simulink model "2_5285361396970701638"  (R2023b)
settings: Solver=VariableStepAuto  StartTime=0.0  StopTime=30  RelTol=1e-3
libraries: simulink x2
settings Model: SimulationMode=accelerator  Creator=ermol  LastModifiedBy=ermol

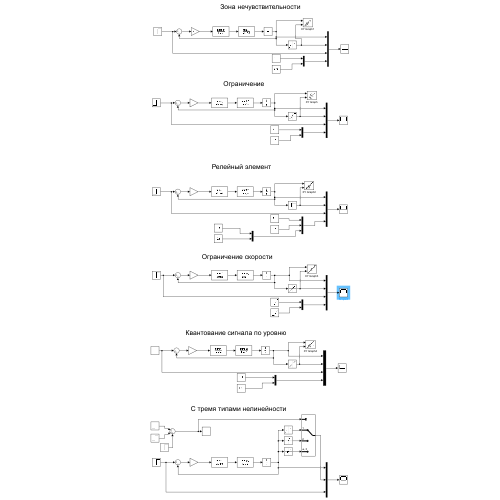
[thumbnail: Simulink's stored preview of the top-level diagram]
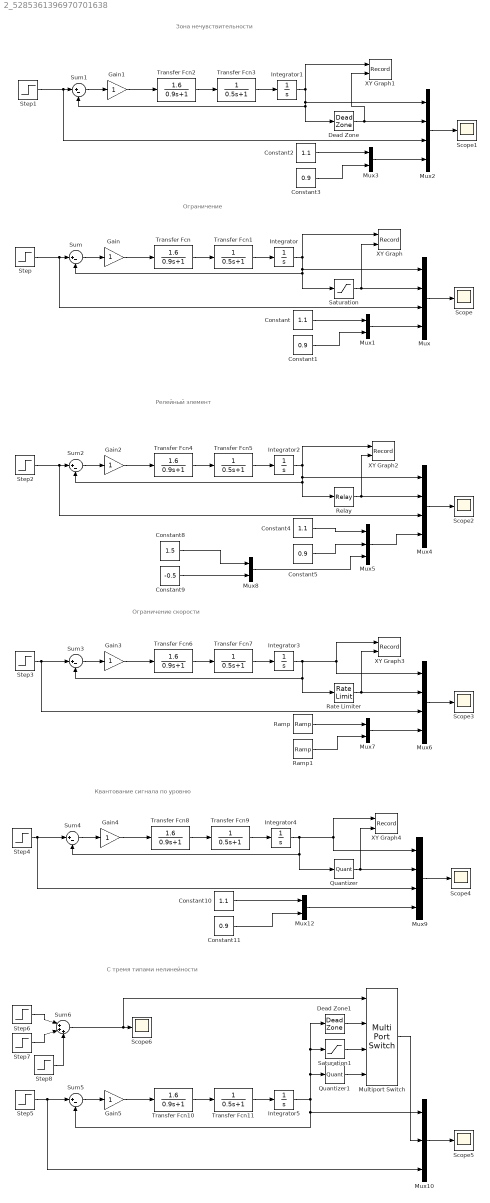
== system 2_5285361396970701638 ==
  note: Ограничение
  note: Зона нечувствительности
  note: Релейный элемент
  note: Ограничение скорости
  note: Квантование сигнала по уровню
  note: С тремя типами нелинейности
  Constant{,2,4,10} (4 alike) : Constant  Value=1.1
  Constant{1,3,5,11} (4 alike) : Constant  Value=0.9
  Constant8 : Constant  Value=1.5
  Constant9 : Constant  Value=-0.5
  Dead Zone : DeadZone  LowerValue=0.9  UpperValue=1.1
  Dead Zone1 : DeadZone  LowerValue=0.9  UpperValue=1.1
  Gain{,1..5} (6 alike) : Gain
  Integrator{,1..5} (6 alike) : Integrator
  Multiport Switch : MultiPortSwitch  SaturateOnIntegerOverflow=off  InputSameDT=off
  Mux{,2,4,6,9} (5 alike) : Mux
  Mux{1,3,7..8,12} (5 alike) : Mux  Inputs=2
  Mux10 : Mux  Inputs=3
  Mux5 : Mux  Inputs=3
  Quantizer : Quantizer  QuantizationInterval=0.2
  Quantizer1 : Quantizer  QuantizationInterval=0.2
  Ramp : simulink/Sources/Ramp  slope=0.3  start=0  InitialOutput=0
  Ramp1 : simulink/Sources/Ramp  slope=-0.15  start=0  InitialOutput=0
  Rate Limiter : RateLimiter  RisingSlewLimit=0.3  FallingSlewLimit=-0.15  SampleTimeMode=inherited
  Relay : Relay  OnSwitchValue=1.1  OffSwitchValue=0.9  OnOutputValue=1.5  OffOutputValue=-0.5
  Saturation : Saturate  UpperLimit=1.1  LowerLimit=0.9
  Saturation1 : Saturate  UpperLimit=1.1  LowerLimit=0.9
  Scope{,1..6} (7 alike) : Scope
  Step{,1..6} (7 alike) : Step  Time=0  SampleTime=0
  Step7 : Step  Time=10  SampleTime=0
  Step8 : Step  Time=20  SampleTime=0
  Sum{,1..5} (6 alike) : Sum  Inputs=|+-
  Sum6 : Sum  Inputs=|+++
  Transfer Fcn{,2,4,6,8,10} (6 alike) : TransferFcn  Numerator=[1.6]  Denominator=[0.9 1]
  Transfer Fcn{1,3,5,7,9,11} (6 alike) : TransferFcn  Denominator=[0.5 1]
  XY Graph : Record  FileSettingsInternal="{\"entries\":[{\"content\":{\"excelSettings\":{\"content\":{},\"type\":\"Streamout.ExcelSettings\"}},\"type\":\"Streamout.FileSettingStorage\",\"uuid\":\"\"}],\"packageUris\":[\"http:\\/\\/schema.mathworks.com\\/mf0\\/streamout_blocks\\/R2020a\"],\"version\":\"1.0\"}"  Layout=[1 1]  SignalsInternal="{\"entries\":[{\"content\":{\"signals\":[{\"content\":{\"blockPath\":[],\"dimensions\":[1],\"domain\":\"\",\"lineColor\":\"#a2142f\",\"plots\":[1],\"port\":1,\"sid\":[\"\"],\"signalID\":2000,\"signalName\":\"Integrator\"},\"type\":\"RecordBlkView.Signal\",\"uuid\":\"\"},{\"content\":{\"blockPath\":[],\"dimensions\":[1],\"domain\":\"\",\"lineColor\":\"#139fff\",\"plots\":[1],\"port\":2,\"sid\":[\"\"],\"signalID\":2004,\"signalName\":\"Saturation\"},\"type\":\"RecordBlkView.Signal\",\"uuid\":\"\"}]},\"type\":\"RecordBlkView.InputSignals\",\"uuid\":\"\"}],\"packageUris\":[\"http:\\/\\/schema.mathworks.com\\/mf0\\/streamout_blocks\\/R2020a\"],\"version\":\"1.0\"}"  VisualizationBindings="{\"xyplotplugin\":{\"info\":[{\"series\":[{\"bindingParametersList\":[{\"parameter\":\"X-Axis\",\"signalID\":2000,\"signalName\":\"Integrator\"},{\"parameter\":\"Y-Axis\",\"signalID\":2004,\"signalName\":\"Saturation\"}],\"seriesID\":16176}],\"subplotID\":1}]}}"  CompatibilityTag=XY
  XY Graph1 : Record  FileSettingsInternal="{\"entries\":[{\"content\":{\"excelSettings\":{\"content\":{},\"type\":\"Streamout.ExcelSettings\"}},\"type\":\"Streamout.FileSettingStorage\",\"uuid\":\"\"}],\"packageUris\":[\"http:\\/\\/schema.mathworks.com\\/mf0\\/streamout_blocks\\/R2020a\"],\"version\":\"1.0\"}"  Layout=[1 1]  SignalsInternal="{\"entries\":[{\"content\":{\"signals\":[{\"content\":{\"blockPath\":[],\"dimensions\":[1],\"domain\":\"\",\"lineColor\":\"#a2142f\",\"plots\":[1],\"port\":1,\"sid\":[\"\"],\"signalID\":2016,\"signalName\":\"Integrator1\"},\"type\":\"RecordBlkView.Signal\",\"uuid\":\"\"},{\"content\":{\"blockPath\":[],\"dimensions\":[1],\"domain\":\"\",\"lineColor\":\"#139fff\",\"plots\":[1],\"port\":2,\"sid\":[\"\"],\"signalID\":2020,\"signalName\":\"Dead Zone\"},\"type\":\"RecordBlkView.Signal\",\"uuid\":\"\"}]},\"type\":\"RecordBlkView.InputSignals\",\"uuid\":\"\"}],\"packageUris\":[\"http:\\/\\/schema.mathworks.com\\/mf0\\/streamout_blocks\\/R2020a\"],\"version\":\"1.0\"}"  VisualizationBindings="{\"xyplotplugin\":{\"info\":[{\"series\":[{\"bindingParametersList\":[{\"parameter\":\"X-Axis\",\"signalID\":2016,\"signalName\":\"Integrator1\"},{\"parameter\":\"Y-Axis\",\"signalID\":2020,\"signalName\":\"Dead Zone\"}],\"seriesID\":41346},{\"bindingParametersList\":[{\"parameter\":\"X-Axis\",\"signalID\":2016,\"signalName\":\"Integrator1\"},{\"parameter\":\"Y-Axis\",\"signalID\":2020,\"signalName\":\"Dead Zone\"}],\"seriesID\":405}],\"subplotID\":1}]}}"  CompatibilityTag=XY
  XY Graph2 : Record  FileSettingsInternal="{\"entries\":[{\"content\":{\"excelSettings\":{\"content\":{},\"type\":\"Streamout.ExcelSettings\"}},\"type\":\"Streamout.FileSettingStorage\",\"uuid\":\"\"}],\"packageUris\":[\"http:\\/\\/schema.mathworks.com\\/mf0\\/streamout_blocks\\/R2020a\"],\"version\":\"1.0\"}"  Layout=[1 1]  SignalsInternal="{\"entries\":[{\"content\":{\"signals\":[{\"content\":{\"blockPath\":[],\"dimensions\":[1],\"domain\":\"\",\"lineColor\":\"#a2142f\",\"plots\":[1],\"port\":1,\"sid\":[\"\"],\"signalID\":2024,\"signalName\":\"Integrator2\"},\"type\":\"RecordBlkView.Signal\",\"uuid\":\"\"},{\"content\":{\"blockPath\":[],\"dimensions\":[1],\"domain\":\"\",\"lineColor\":\"#139fff\",\"plots\":[1],\"port\":2,\"sid\":[\"\"],\"signalID\":2028,\"signalName\":\"Relay\"},\"type\":\"RecordBlkView.Signal\",\"uuid\":\"\"}]},\"type\":\"RecordBlkView.InputSignals\",\"uuid\":\"\"}],\"packageUris\":[\"http:\\/\\/schema.mathworks.com\\/mf0\\/streamout_blocks\\/R2020a\"],\"version\":\"1.0\"}"  VisualizationBindings="{\"xyplotplugin\":{\"info\":[{\"series\":[{\"bindingParametersList\":[{\"parameter\":\"X-Axis\",\"signalID\":2024,\"signalName\":\"Integrator2\"},{\"parameter\":\"Y-Axis\",\"signalID\":2028,\"signalName\":\"Relay\"}],\"seriesID\":26503},{\"bindingParametersList\":[{\"parameter\":\"X-Axis\",\"signalID\":2028,\"signalName\":\"Relay\"}],\"seriesID\":436}],\"subplotID\":1}]}}"  CompatibilityTag=XY
  XY Graph3 : Record  FileSettingsInternal="{\"entries\":[{\"content\":{\"excelSettings\":{\"content\":{},\"type\":\"Streamout.ExcelSettings\"}},\"type\":\"Streamout.FileSettingStorage\",\"uuid\":\"\"}],\"packageUris\":[\"http:\\/\\/schema.mathworks.com\\/mf0\\/streamout_blocks\\/R2020a\"],\"version\":\"1.0\"}"  Layout=[1 1]  SignalsInternal="{\"entries\":[{\"content\":{\"signals\":[{\"content\":{\"blockPath\":[],\"dimensions\":[1],\"domain\":\"\",\"lineColor\":\"#a2142f\",\"plots\":[1],\"port\":1,\"sid\":[\"\"],\"signalID\":2032,\"signalName\":\"Integrator3\"},\"type\":\"RecordBlkView.Signal\",\"uuid\":\"\"},{\"content\":{\"blockPath\":[],\"dimensions\":[1],\"domain\":\"\",\"lineColor\":\"#139fff\",\"plots\":[1],\"port\":2,\"sid\":[\"\"],\"signalID\":2036,\"signalName\":\"Rate Limiter\"},\"type\":\"RecordBlkView.Signal\",\"uuid\":\"\"}]},\"type\":\"RecordBlkView.InputSignals\",\"uuid\":\"\"}],\"packageUris\":[\"http:\\/\\/schema.mathworks.com\\/mf0\\/streamout_blocks\\/R2020a\"],\"version\":\"1.0\"}"  VisualizationBindings="{\"xyplotplugin\":{\"info\":[{\"series\":[{\"bindingParametersList\":[{\"parameter\":\"X-Axis\",\"signalID\":2032,\"signalName\":\"Integrator3\"},{\"parameter\":\"Y-Axis\",\"signalID\":2036,\"signalName\":\"Rate Limiter\"}],\"seriesID\":45437},{\"bindingParametersList\":[{\"parameter\":\"X-Axis\",\"signalID\":2036,\"signalName\":\"Rate Limiter\"}],\"seriesID\":436}],\"subplotID\":1}]}}"  CompatibilityTag=XY
  XY Graph4 : Record  FileSettingsInternal="{\"entries\":[{\"content\":{\"excelSettings\":{\"content\":{},\"type\":\"Streamout.ExcelSettings\"}},\"type\":\"Streamout.FileSettingStorage\",\"uuid\":\"\"}],\"packageUris\":[\"http:\\/\\/schema.mathworks.com\\/mf0\\/streamout_blocks\\/R2020a\"],\"version\":\"1.0\"}"  Layout=[1 1]  SignalsInternal="{\"entries\":[{\"content\":{\"signals\":[{\"content\":{\"blockPath\":[],\"dimensions\":[1],\"domain\":\"\",\"lineColor\":\"#a2142f\",\"plots\":[1],\"port\":1,\"sid\":[\"\"],\"signalID\":2008,\"signalName\":\"Integrator4\"},\"type\":\"RecordBlkView.Signal\",\"uuid\":\"\"},{\"content\":{\"blockPath\":[],\"dimensions\":[1],\"domain\":\"\",\"lineColor\":\"#139fff\",\"plots\":[1],\"port\":2,\"sid\":[\"\"],\"signalID\":2012,\"signalName\":\"Quantizer\"},\"type\":\"RecordBlkView.Signal\",\"uuid\":\"\"}]},\"type\":\"RecordBlkView.InputSignals\",\"uuid\":\"\"}],\"packageUris\":[\"http:\\/\\/schema.mathworks.com\\/mf0\\/streamout_blocks\\/R2020a\"],\"version\":\"1.0\"}"  VisualizationBindings="{\"xyplotplugin\":{\"info\":[{\"series\":[{\"bindingParametersList\":[{\"parameter\":\"X-Axis\",\"signalID\":2008,\"signalName\":\"Integrator4\"},{\"parameter\":\"Y-Axis\",\"signalID\":2012,\"signalName\":\"Quantizer\"}],\"seriesID\":47889},{\"bindingParametersList\":[{\"parameter\":\"X-Axis\",\"signalID\":2012,\"signalName\":\"Quantizer\"}],\"seriesID\":436}],\"subplotID\":1}]}}"  CompatibilityTag=XY
  wires:
  Sum/1 -> Gain/1
  Step/1 -> Mux/3, Sum/1
  Gain/1 -> Transfer Fcn/1
  Transfer Fcn/1 -> Transfer Fcn1/1
  Transfer Fcn1/1 -> Integrator/1
  Integrator/1 -> Saturation/1, Sum/2, Mux/1, XY Graph/1
  Mux/1 -> Scope/1
  Mux1/1 -> Mux/4
  Constant/1 -> Mux1/1
  Constant1/1 -> Mux1/2
  Saturation/1 -> XY Graph/2, Mux/2
  Constant2/1 -> Mux3/1
  Constant3/1 -> Mux3/2
  Dead Zone/1 -> XY Graph1/2, Mux2/2
  Mux3/1 -> Mux2/4
  Gain1/1 -> Transfer Fcn2/1
  Step1/1 -> Mux2/3, Sum1/1
  Sum1/1 -> Gain1/1
  Integrator1/1 -> Dead Zone/1, Sum1/2, Mux2/1, XY Graph1/1
  Transfer Fcn2/1 -> Transfer Fcn3/1
  Transfer Fcn3/1 -> Integrator1/1
  Mux2/1 -> Scope1/1
  Transfer Fcn4/1 -> Transfer Fcn5/1
  Integrator2/1 -> Relay/1, Sum2/2, Mux4/1, XY Graph2/1
  Mux4/1 -> Scope2/1
  Sum2/1 -> Gain2/1
  Step2/1 -> Mux4/3, Sum2/1
  Mux5/1 -> Mux4/4
  Relay/1 -> XY Graph2/2, Mux4/2
  Gain2/1 -> Transfer Fcn4/1
  Constant5/1 -> Mux5/2
  Transfer Fcn5/1 -> Integrator2/1
  Constant4/1 -> Mux5/1
  Ramp/1 -> Mux7/1
  Mux7/1 -> Mux6/4
  Transfer Fcn7/1 -> Integrator3/1
  Ramp1/1 -> Mux7/2
  Rate Limiter/1 -> XY Graph3/2, Mux6/2
  Step3/1 -> Mux6/3, Sum3/1
  Gain3/1 -> Transfer Fcn6/1
  Sum3/1 -> Gain3/1
  Transfer Fcn6/1 -> Transfer Fcn7/1
  Mux6/1 -> Scope3/1
  Integrator3/1 -> Rate Limiter/1, Sum3/2, Mux6/1, XY Graph3/1
  Constant8/1 -> Mux8/1
  Mux8/1 -> Mux5/3
  Constant9/1 -> Mux8/2
  Gain4/1 -> Transfer Fcn8/1
  Mux9/1 -> Scope4/1
  Integrator4/1 -> Quantizer/1, Sum4/2, Mux9/1, XY Graph4/1
  Transfer Fcn8/1 -> Transfer Fcn9/1
  Quantizer/1 -> XY Graph4/2, Mux9/2
  Step4/1 -> Mux9/3, Sum4/1
  Transfer Fcn9/1 -> Integrator4/1
  Sum4/1 -> Gain4/1
  Integrator5/1 -> Dead Zone1/1, Saturation1/1, Quantizer1/1, Sum5/2, Mux10/1
  Step5/1 -> Mux10/3, Sum5/1
  Sum5/1 -> Gain5/1
  Transfer Fcn11/1 -> Integrator5/1
  Gain5/1 -> Transfer Fcn10/1
  Mux10/1 -> Scope5/1
  Transfer Fcn10/1 -> Transfer Fcn11/1
  Step6/1 -> Sum6/1
  Step7/1 -> Sum6/2
  Step8/1 -> Sum6/3
  Sum6/1 -> Multiport Switch/1, Scope6/1
  Dead Zone1/1 -> Multiport Switch/2
  Saturation1/1 -> Multiport Switch/3
  Quantizer1/1 -> Multiport Switch/4
  Multiport Switch/1 -> Mux10/2
  Constant10/1 -> Mux12/1
  Constant11/1 -> Mux12/2
  Mux12/1 -> Mux9/4
